simulink model "Rosseler_Simulink"  (R2020a)
settings: Solver=VariableStepAuto  StartTime=0.0  StopTime=250  RelTol=1e-3
settings Model: Creator=User  LastModifiedBy=User

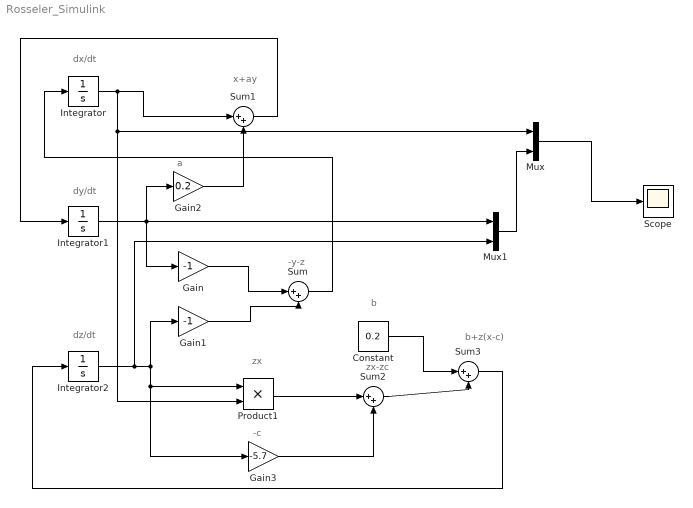
== system Rosseler_Simulink ==
  note: b+z(x-c)
  note: zx-zc
  note: -c
  note: zx
  note: b
  note: x+ay
  note: a
  note: -y-z
  note: dz/dt
  note: dy/dt
  note: dx/dt
  Constant : Constant  Value=0.2
  Gain : Gain  Gain=-1
  Gain1 : Gain  Gain=-1
  Gain2 : Gain  Gain=0.2
  Gain3 : Gain  Gain=-5.7
  Integrator : Integrator  InitialCondition=2.01
  Integrator1 : Integrator  InitialCondition=3.1
  Integrator2 : Integrator  InitialCondition=8.2
  Mux : Mux  Inputs=2
  Mux1 : Mux  Inputs=2
  Product1 : Product
  Scope : Scope
  Sum{,1..3} (4 alike) : Sum  Inputs=|++
  wires:
  Integrator2/1 -> Mux1/2, Gain3/1, Product1/1, Gain1/1
  Integrator1/1 -> Gain2/1, Mux1/1, Gain/1
  Gain1/1 -> Sum/2
  Gain/1 -> Sum/1
  Sum/1 -> Integrator/1
  Gain2/1 -> Sum1/2
  Integrator/1 -> Product1/2, Mux/1, Sum1/1
  Sum1/1 -> Integrator1/1
  Gain3/1 -> Sum2/2
  Product1/1 -> Sum2/1
  Sum2/1 -> Sum3/2
  Constant/1 -> Sum3/1
  Sum3/1 -> Integrator2/1
  Mux1/1 -> Mux/2
  Mux/1 -> Scope/1
